simulink model "TwoTank_Linearization"  (R2021a)
settings: Solver=VariableStepAuto  StartTime=0.0  StopTime=1200  RelTol=1e-3
values from neighbouring files (symbols this model uses):
  h1_bar = x_bar(1)    [main_LQ.m]
  h2_bar = (a1 / (S1 * k))^2 * h1_ref    [compute_equilibrium.m]    (also in main_LQ.m = x_bar(2))
  q_bar = u_bar    [main_LQ.m]
libraries: simulink x1
settings Model: Creator=fabio  LastModifiedBy=fabio
settings SolverCC: AlgebraicLoopSolver=TrustRegion
settings OptimizationCC: BlockReduction=off  DefaultParameterBehavior=Inlined  BufferReuse=off
settings DebuggingCC: SFMachineParentedDataDiag=warning

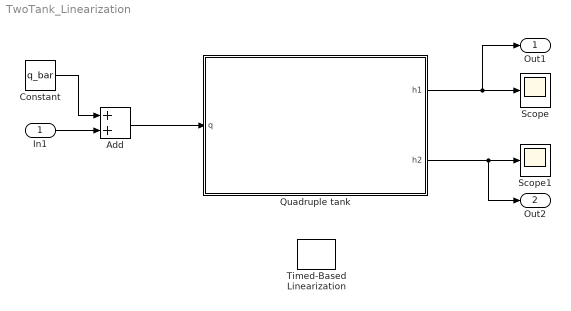
== system TwoTank_Linearization ==
  In1 : Inport
  Add : Sum
  Constant : Constant  Value=q_bar
  Quadruple tank : Subsystem  mask{h_0=[ h1_bar, h2_bar], At=[1.31e-4, 9.27e-5], S=[0.06, 0.06], gamma=0.4, enable_saturation=on, enable_rate=off}
      mask prompts: h_0 "Initial level"; At "Tank discharge constant"; S "Tank section"; gamma "Valve split coefficient"; enable_saturation "Control saturation"; enable_rate "Control rate limit"
      mask DialogControl h_0 Tooltip: [cm]
      mask DialogControl At Tooltip: [cm^2]
      mask DialogControl S Tooltip: [cm^2]
      mask DialogControl gamma Tooltip: [cm/s^2]
      mask Display:
      | disp('Quadruple\nTank');
      | port_label('input', 1, 'q', 'interpreter', 'tex');
      | port_label('output', 1, 'h_1', 'interpreter', 'tex');
      | port_label('output', 2, 'h_2', 'interpreter', 'tex');
  Scope : Scope
  Scope1 : Scope
  Timed-Based Linearization : simulink/Model-Wide Utilities/Timed-Based Linearization  LinearizationTime=1  SampleTime=0
      settings: SourceProductBaseCode=SL
  Out1 : Outport
  Out2 : Outport  Port=2
  wires:
  Quadruple tank/1(h1) -> Out1/1, Scope/1
  Quadruple tank/2(h2) -> Out2/1, Scope1/1
  Constant/1 -> Add/1
  Add/1 -> Quadruple tank/1(q)
  In1/1 -> Add/2

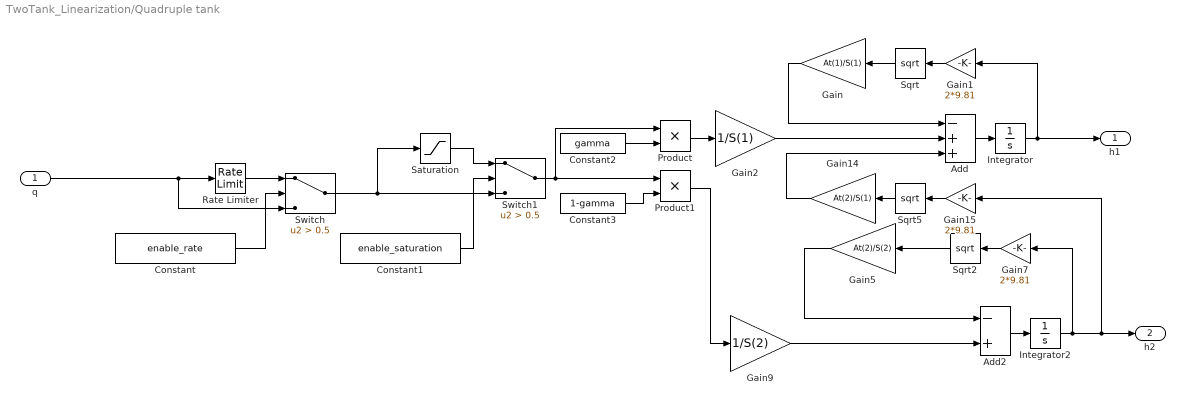
== system TwoTank_Linearization/Quadruple tank ==
  q : Inport
  Add : Sum  Inputs=-++
  Add2 : Sum  Inputs=-+
  Constant : Constant  Value=enable_rate
  Constant1 : Constant  Value=enable_saturation
  Constant2 : Constant  Value=gamma
  Constant3 : Constant  Value=1-gamma
  Gain : Gain  Gain=At(1)/S(1)
  Gain1 : Gain  Gain=2*9.81
  Gain14 : Gain  Gain=At(2)/S(1)
  Gain15 : Gain  Gain=2*9.81
  Gain2 : Gain  Gain=1/S(1)
  Gain5 : Gain  Gain=At(2)/S(2)
  Gain7 : Gain  Gain=2*9.81
  Gain9 : Gain  Gain=1/S(2)
  Integrator : Integrator  InitialCondition=h_0(1)  LimitOutput=on  UpperSaturationLimit=1.3  LowerSaturationLimit=0
  Integrator2 : Integrator  InitialCondition=h_0(2)  LimitOutput=on  UpperSaturationLimit=1.2  LowerSaturationLimit=0
  Product : Product
  Product1 : Product
  Rate Limiter : RateLimiter  SampleTimeMode=inherited  LinearizeAsGain=off
  Saturation : Saturate  UpperLimit=1e-3  LowerLimit=1e-4  LinearizeAsGain=off
  Sqrt : Sqrt  SaturateOnIntegerOverflow=on
  Sqrt2 : Sqrt  SaturateOnIntegerOverflow=on
  Sqrt5 : Sqrt  SaturateOnIntegerOverflow=on
  Switch : Switch  Criteria=u2 > Threshold  Threshold=0.5
  Switch1 : Switch  Criteria=u2 > Threshold  Threshold=0.5
  h1 : Outport
  h2 : Outport  Port=2
  wires:
  Integrator/1 -> Gain1/1, h1/1
  Add/1 -> Integrator/1
  Gain1/1 -> Sqrt/1
  Sqrt/1 -> Gain/1
  Gain/1 -> Add/1
  Gain2/1 -> Add/2
  Product/1 -> Gain2/1
  Add2/1 -> Integrator2/1
  Gain7/1 -> Sqrt2/1
  Sqrt2/1 -> Gain5/1
  Gain9/1 -> Add2/2
  Product1/1 -> Gain9/1
  Gain15/1 -> Sqrt5/1
  Sqrt5/1 -> Gain14/1
  Integrator2/1 -> Gain7/1, Gain15/1, h2/1
  Gain14/1 -> Add/3
  Gain5/1 -> Add2/1
  Constant2/1 -> Product/2
  Constant3/1 -> Product1/2
  Rate Limiter/1 -> Switch/1
  q/1 -> Switch/3, Rate Limiter/1
  Constant/1 -> Switch/2
  Saturation/1 -> Switch1/1
  Switch/1 -> Saturation/1, Switch1/3
  Constant1/1 -> Switch1/2
  Switch1/1 -> Product1/1, Product/1
